simulink model "frequency_resolution"  (Simulink 6.6)
settings: Solver=VariableStepDiscrete  SolverMode=SingleTasking  StartTime=0.0  StopTime=18*2048/100e3  RelTol=1e-3
undefined symbols (not defined in the file): get
libraries: xbsIndex_r4 x7, dspsnks4 x1, simulink x1
settings Model: Creator=lcrockett  LastModifiedBy=lcrockett
settings DataIOCC: SignalLoggingName=sigsOut
settings OptimizationCC: InlineParams=on  InlineInvariantSignals=on
settings DebuggingCC: SignalResolutionControl=TryResolveAllWithWarning  SolverPrmCheckMsg=none  MultiTaskDSMMsg=warning  MultiTaskCondExecSysMsg=none  StrictBusMsg=None
settings HardwareCC: TargetUnknown=on
settings RTWCC: IncludeERTFirstTime=on
settings GRTTargetCC: ModelReferenceCompliant=off  MatFileLogging=off

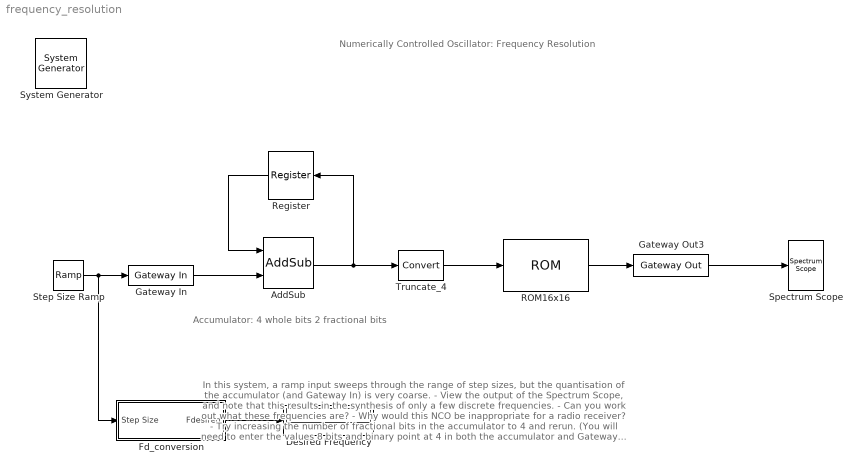
== system frequency_resolution ==
  note: Numerically Controlled Oscillator:
      | Frequency Resolution
  note: Accumulator:
      | 4 whole bits
      | 2 fractional bits
  note: In this system, a ramp input sweeps through the range of step sizes,
      | but the quantisation of the accumulator (and Gateway In) is very coarse.
      | - View the output of the Spectrum Scope, and note that this results
      |   in the synthesis of only a few discrete frequencies.
      | - Can you work out what these frequencies are?
      |  - Why would this NCO be inappropriate for a radio receiver?
      | - Try increasing the number of fractional bits in the accumulator  to 4
      |   and rerun. (You will need to enter the values 8 bits and binary point
      |   at 4 in both the accumulator and Gateway In blocks). What do you
      |   see now?
  " System Generator" : xbsIndex_r4/ System Generator  Tag=genX  SystemSampleTime=-1  xilinxfamily=virtex2  part=xc2v40  speed=-4  package=cs144  synthesis_tool=XST  clock_wrapper=Clock Enables  directory=./netlist  testbench=off  simulink_period=1/100e3  sysclk_period=50  dcm_input_clock_period=100  incr_netlist=off  trim_vbits=Everywhere in SubSystem  dbl_ovrd=No Where in SubSystem  core_generation=According to Block Masks  run_coregen=off  deprecated_control=off  eval_field=0  block_type=sysgen
      settings: block_version=9.1.01
  AddSub : xbsIndex_r4/AddSub  mode=Addition  use_carryin=off  use_carryout=off  en=off  latency=0  precision=User Defined  arith_type=Unsigned  n_bits=6  bin_pt=2  quantization=Truncate  overflow=Wrap  dbl_ovrd=off  use_behavioral_HDL=on  pipelined=off  use_rpm=on  block_type=addsub
      settings: xl_area=[5 0 0 10 0 0 0]  block_version=VER_STRING_GOES_HERE
  Desired Frequency : Display
  Fd_conversion : Subsystem
  Gateway In : xbsIndex_r4/Gateway In  arith_type=Unsigned  n_bits=6  bin_pt=2  quantization="Round  (unbiased: +/- Inf)"  overflow=Wrap  period=1/100e+3  dbl_ovrd=off  timing_constraint=None  locs_specified=off  LOCs={}  block_type=gatewayin
      settings: infoedit="Gateway in block.  Converts inputs of type Simulink integer, double and fixed point to  Xilinx fixed point type.<P><P>Hardware notes:  In hardware these blocks become top level input ports."
  Gateway Out3 : xbsIndex_r4/Gateway Out  hdl_port=on  timing_constraint=None  locs_specified=off  LOCs={}  block_type=gatewayout
      settings: infoedit="Gateway out block.  Converts Xilinx fixed point inputs into ouputs of type Simulink integer, double, or fixed point.<P><P>Hardware notes:  In hardware these blocks become top level output ports or are discarded, depending on how they are configured."  xl_area=[0 0 0 0 16 0 0]  block_version=VER_STRING_GOES_HERE
  ROM16x16 : xbsIndex_r4/ROM  depth=16  initVector=sin(pi*(0:15)/8)  distributed_mem=Block RAM  rst=off  init_reg=0  en=off  latency=1  arith_type="Signed  (2's comp)"  n_bits=16  bin_pt=15  dbl_ovrd=off  optimize=Area  use_rpm=off  block_type=sprom
      settings: xl_area=[8 16 0 16 0 0 0]  block_version=VER_STRING_GOES_HERE
  Register : xbsIndex_r4/Register  Orientation=left  init=0  rst=off  en=off  dbl_ovrd=off  block_type=register
      settings: xl_area=[5 10 0 0 0 0 0]  block_version=VER_STRING_GOES_HERE
  Spectrum Scope : dspsnks4/Spectrum Scope  DialogController=dspdialog.SpectrumScope  DialogControllerArgs=DataTag1  SystemSampleTime=-1  ScopeProperties=on  Domain=Frequency  HorizSpan=1  UseBuffer=on  BufferSize=128  Overlap=64  inpFftLenInherit=on  FFTlength=128  numAvg=2  DisplayProperties=off  AxisGrid=on  Memory=off  FrameNumber=on  AxisLegend=off  AxisZoom=off  OpenScopeAtSimStart=on  OpenScopeImmediately=off  FigPos=get(0,'defaultfigureposition')  AxisProperties=off  XUnits=Hertz  XRange=[0...Fs/2]  InheritXIncr=on  XIncr=1.0  XLabel=Samples  XLimit=Auto  YUnits=dB  XMax=1  XMin=0  YLabel=Magnitude-squared, dB  LineProperties=off  wintypeSpecScope=Hann  RsSpecScope=50  betaSpecScope=5  winsampSpecScope=Periodic
      settings: YMin=-10  YMax=15
  Step Size Ramp : simulink/Sources/Ramp  SystemSampleTime=-1  slope=20  start=0  X0=0
  Truncate_4 : xbsIndex_r4/Convert  arith_type=Unsigned  n_bits=4  bin_pt=0  quantization="Round  (unbiased: +/- Inf)"  overflow=Wrap  latency=0  dbl_ovrd=off  pipeline=off  block_type=convert
      settings: xl_area=[2 0 0 4 0 0 0]  block_version=VER_STRING_GOES_HERE
  wires:
  AddSub/1 -> Register/1, Truncate_4/1
  Register/1 -> AddSub/1
  Truncate_4/1 -> ROM16x16/1
  ROM16x16/1 -> Gateway Out3/1
  Gateway Out3/1 -> Spectrum Scope/1
  Gateway In/1 -> AddSub/2
  Step Size Ramp/1 -> Gateway In/1, Fd_conversion/1(Step Size)
  Fd_conversion/1(Fdesired) -> Desired Frequency/1

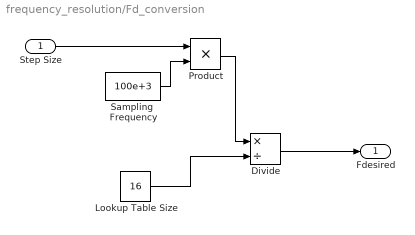
== system frequency_resolution/Fd_conversion ==
  Step Size : Inport
  Divide : Product  Inputs=*/  OutScaling=2^-10
  Lookup Table Size : Constant  Value=16
  Product : Product  RndMeth=Zero
  Sampling  Frequency : Constant  Value=100e+3
  Fdesired : Outport
  wires:
  Sampling  Frequency/1 -> Product/2
  Product/1 -> Divide/1
  Lookup Table Size/1 -> Divide/2
  Step Size/1 -> Product/1
  Divide/1 -> Fdesired/1
